simulink library "lib_Convection_Sutherland"  (R2015a)
settings: Solver=ode45  StartTime=0.0  StopTime=10.0  RelTol=1e-3
settings Model: Creator=jlkratz  LastModifiedBy=jlkratz

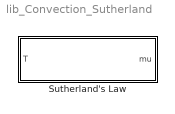
== system lib_Convection_Sutherland ==
  Sutherland's Law : Subsystem  mask(TSAT: Sutherland's Law){Tref_M=524.07, muref_M=3.8157*10^-7, S_M=216.2162}
      mask prompts: Tref_M "Tref_M - Reference temperature"; muref_M "muref_M - Reference viscosity (viscosity at the reference temperature)"; S_M "S_M - The Sutherland temperature"
      mask help:
      | This block implements Sutherlands law to approximate viscosity of a gas. Given appropriate parameters it is applicable to various gases. Sutherland's law is based on kinematic theory of ideal gases and an idealized intermolecular-force potential. It typically gives results that are accurate within a few percent over a wide temperature range. The temperature range in which the equation is valid will be dependent on the gas and the paramters you are using. Be sure to observe the valid temperature range when using this block to assure accurate results. Units of the temperature and viscosity will be dependent on the units of the parameters chosen which should be consistent.
      |
      | Some values of parameters for common gases can be found in the help menu of this block.
      mask Help: web(which('Convection_TSAT_SutherlandsLaw.html'),'-helpbrowser')

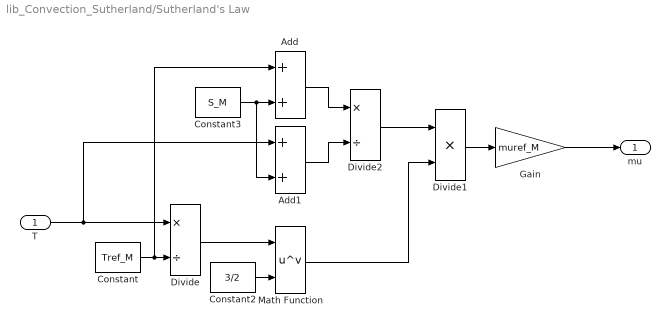
== system lib_Convection_Sutherland/Sutherland's Law ==
  T : Inport
  Add : Sum
  Add1 : Sum
  Constant : Constant  Value=Tref_M
  Constant2 : Constant  Value=3/2
  Constant3 : Constant  Value=S_M
  Divide : Product  Inputs=*/
  Divide1 : Product  Inputs=**
  Divide2 : Product  Inputs=*/
  Gain : Gain  Gain=muref_M
  Math Function : Math  Operator=pow  SaturateOnIntegerOverflow=on
  mu : Outport
  wires:
  Add1/1 -> Divide2/2
  Constant/1 -> Divide/2, Add/1
  Divide1/1 -> Gain/1
  Constant2/1 -> Math Function/2
  Add/1 -> Divide2/1
  Math Function/1 -> Divide1/2
  T/1 -> Divide/1, Add1/1
  Constant3/1 -> Add/2, Add1/2
  Divide/1 -> Math Function/1
  Divide2/1 -> Divide1/1
  Gain/1 -> mu/1
